simulink model "boost_converter"  (R2014b)
settings: Solver=ode23  StartTime=0.0  StopTime=0.5  MaxStep=1e-4  RelTol=1e-3
libraries: powerlib x12
settings Model: Creator=Amr Saleh  LastModifiedBy=Amr Saleh

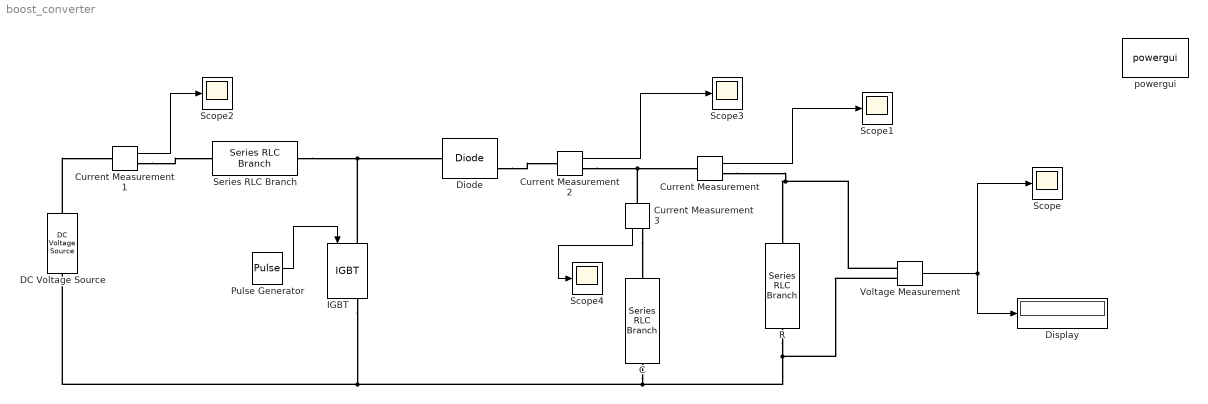
== system boost_converter ==
  C : powerlib/Elements/Series RLC Branch  LConnTagsString=__new0  RConnTagsString=__new0  BranchType=C  Resistance=1  Inductance=1e-3  SetiL0=off  InitialCurrent=0  Capacitance=32e-6  Setx0=off  InitialVoltage=0  Measurements=None
  Current Measurement{,1..3} (4 alike) : powerlib/Measurements/Current Measurement  PhasorSimulation=off  OutputType=Complex  PSBequivalent=0
  DC Voltage Source : powerlib/Electrical Sources/DC Voltage Source  Amplitude=20  Measurements=None
  Diode : powerlib/Power Electronics/Diode  Ron=0.0001  Lon=0  Vf=0.5  IC=0  UseSnubber=off  Rs=500  Cs=250e-9  Measurements=on
  Display : Display
  IGBT : powerlib/Power Electronics/IGBT  Ron=0.0001  Lon=0  Vf=0.5  Tf=1e-6  Tt=2e-6  IC=0  Rs=1e5  Cs=inf  Measurements=on
  Pulse Generator : DiscretePulseGenerator  PulseType=Time based  Period=1/5000  PulseWidth=80
  R : powerlib/Elements/Series RLC Branch  LConnTagsString=__new0  RConnTagsString=__new0  BranchType=R  Resistance=100  Inductance=1e-3  SetiL0=off  InitialCurrent=0  Capacitance=1e-6  Setx0=off  InitialVoltage=0  Measurements=None
  Scope{,1..4} (5 alike) : Scope
      Scope settings: YMin=0  YMax=150
      Scope1 settings: YMin=0  YMax=1.5
      Scope2 settings: YMin=0  YMax=10  SaveName=ScopeData2
      Scope3 settings: YMin=0  YMax=1.5  SaveName=ScopeData3
      Scope4 settings: YMin=0  YMax=1.5  SaveName=ScopeData4
  Series RLC Branch : powerlib/Elements/Series RLC Branch  LConnTagsString=__new0  RConnTagsString=__new0  BranchType=L  Resistance=1  Inductance=32e-3  SetiL0=off  InitialCurrent=0  Capacitance=1e-6  Setx0=off  InitialVoltage=0  Measurements=None
  Voltage Measurement : powerlib/Measurements/Voltage Measurement  PhasorSimulation=off  OutputType=Complex  PSBequivalent=0
  powergui : powerlib/powergui  Priority=1  SimulationMode=Continuous  SolverType=Tustin/Backward Euler (TBE)  SampleTime=50e-6  frequency=60  SPID=off  DisableSnubberDevices=off  DisableRonSwitches=off  DisableVfSwitches=off  SwTol=0  DisplayEquations=off  Interpol=off  methode=off  Ts=100  frequencyindice=0  Pbase=100e6  ErrMax=1e-4  Iterations=50  UnitsV=kV  UnitsW=MW  FunctionMessages=off  echomessages=off  HookPort=off  EnableUseOfTLC=off  x0status=blocks  RestoreLinks=warning  ResistiveCurrentMeasurement=off  Frange=[0:2:500]  Ylog=off  Xlog=on  ShowGrid=off  save=off  variable=ZData  structure=0  ZoomFFT=off  StartTime=0.0  cycles=1  DisplayStyle=1  fundamental=60  FreqAxis=off  MaxFrequency=1000  frequencyindicesteady=1  RmsSteady=1  display=off
  wires:
  Voltage Measurement/1 -> Scope/1, Display/1
  Pulse Generator/1 -> IGBT/1
  Current Measurement/1 -> Scope1/1
  Current Measurement1/1 -> Scope2/1
  Current Measurement2/1 -> Scope3/1
  Current Measurement3/1 -> Scope4/1
  connections:
  Series RLC Branch/RConn1 -- IGBT/LConn1 -- Diode/LConn1
  Voltage Measurement/LConn1 -- Current Measurement/RConn1 -- R/RConn1
  R/LConn1 -- Voltage Measurement/LConn2 -- C/LConn1 -- IGBT/RConn1 -- DC Voltage Source/LConn1
  DC Voltage Source/RConn1 -- Current Measurement1/LConn1
  Current Measurement1/RConn1 -- Series RLC Branch/LConn1
  Current Measurement2/RConn1 -- Current Measurement3/LConn1 -- Current Measurement/LConn1
  Diode/RConn1 -- Current Measurement2/LConn1
  Current Measurement3/RConn1 -- C/RConn1
